simulink model "mass_spring_damper_simulink"  (R2022a)
settings: Solver=ode45  StartTime=0.0  StopTime=Sim_Time  MaxStep=0.01  RelTol=1e-3  EnableMultiTasking=on
undefined symbols (not defined in the file): b, F, k, M
settings Model: Creator=dzr3qn  LastModifiedBy=Dr. Ryan Aly
settings SolverCC: AlgebraicLoopSolver=TrustRegion
settings DataIOCC: LimitDataPoints=on  SaveFormat=Array  ReturnWorkspaceOutputs=off
settings OptimizationCC: LifeSpan=inf
settings DebuggingCC: SolverPrmCheckMsg=warning  UnconnectedInputMsg=warning  UnconnectedOutputMsg=warning  UnconnectedLineMsg=warning  SFUnexpectedBacktrackingDiag=warning  SFNoUnconditionalDefaultTransitionDiag=warning  SFExecutionAtInitializationDiag=none  SFMachineParentedDataDiag=warning  ArithmeticOperatorsInVariantConditions=warning
settings HardwareCC: ProdBitPerPointer=32  ProdBitPerSizeT=32  ProdBitPerPtrDiffT=32  ProdLargestAtomicFloat=None  ProdIntDivRoundTo=Undefined  ProdEndianess=Unspecified  ProdWordSize=32  ProdHWDeviceType=32-bit Generic
settings ModelReferenceCC: PropagateSignalLabelsOutOfModel=off
settings SFSimCC: SimUseLocalCustomCode=off  CustomCodeUndefinedFunction=UseInterfaceOnly
settings RTWCC: RTWUseLocalCustomCode=off
settings CodeAppCC: StateflowObjectComments=on
settings GRTTargetCC: TargetLangStandard=C89/C90 (ANSI)
settings ConfigComp: CovMetricSettings=dw  CovSaveCumulativeToWorkspaceVar=on  CovSaveSingleToWorkspaceVar=on  CovExternalEMLEnable=off  CovSFcnEnable=off

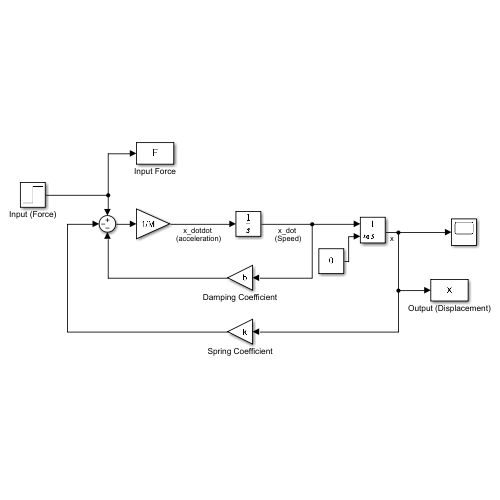
[thumbnail: Simulink's stored preview of the top-level diagram]
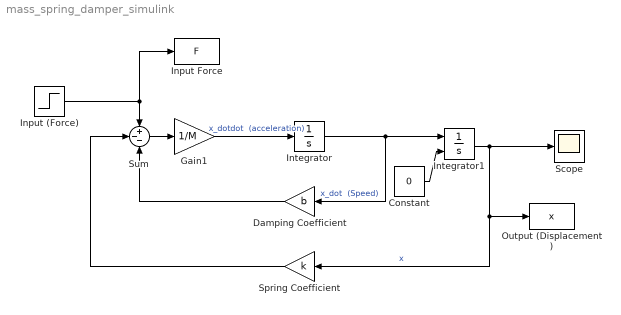
== system mass_spring_damper_simulink ==
  Constant : Constant  Value=0
  Damping Coefficient : Gain  Gain=b
  Gain1 : Gain  Gain=1/M
  Input (Force) : Step  Time=0  After=F  SampleTime=0
  Input Force : ToWorkspace  VariableName=F  SaveFormat=Timeseries  SampleTime=-1
  Integrator : Integrator
  Integrator1 : Integrator  InitialConditionSource=external
  Output (Displacement) : ToWorkspace  VariableName=x  SaveFormat=Timeseries  SampleTime=-1
  Scope : Scope
  Spring Coefficient : Gain  Gain=k
  Sum : Sum  Inputs=+--
  wires:
  Integrator/1 -> Damping Coefficient/1, Integrator1/1  "x_dot  (Speed)"
  Integrator1/1 -> Scope/1, Output (Displacement)/1, Spring Coefficient/1  "x"
  Sum/1 -> Gain1/1
  Gain1/1 -> Integrator/1  "x_dotdot  (acceleration)"
  Damping Coefficient/1 -> Sum/3
  Spring Coefficient/1 -> Sum/2
  Input (Force)/1 -> Input Force/1, Sum/1
  Constant/1 -> Integrator1/2
